simulink model "sim_main_esb_2"  (R2018b)
settings: Solver=VariableStepAuto  StartTime=0.0  StopTime=10  RelTol=1e-3
values from neighbouring files (symbols this model uses):
  A = 0.914    [KALMAN.m]    (also in main_cntl.m = eval(A_eq); main_sys.m = double(A_lin); main_sys_klm.m = double(A_lin); main_tf_0.m = A)
  B = 0.25    [KALMAN.m]    (also in main_cntl.m = eval(B_eq); main_sys.m = double(B_lin); main_sys_klm.m = double(B_lin); main_tf_1.m = eval(B))
  bm = 0.4e-3    (= 0.0004)    [main_cntl.m]    (also in main_sys.m = 0.00047698; main_sys_klm.m = 0.00047698; main_tf_1.m; main_tf_10.m = 0.00047698)
  C = 0.344    [KALMAN.m]    (also in main_sys.m = double( subs( C) ); main_sys_klm.m = double( subs( C) ); main_tf_0.m = [ 0 , 0  , Ks , ds , -Ks , -ds, 0 ]; main_tf_1.m = C_mes)
  D = zeros(7,2)    [main_sys.m]    (also in main_sys_klm.m = zeros(2,2); main_tf_0.m = [ 0 , 0 ]; main_tf_1.m = zeros(1,1); main_tf_10.m = zeros(2,2))
  dg = 0.65    [main_cntl.m]    (also in main_sys.m; main_sys_klm.m; main_tf_1.m; main_tf_10.m)
  dgs = 6    [main_cntl.m]    (also in main_sys.m; main_sys_klm.m; main_tf_1.m; main_tf_10.m)
  J_act = [0.000306 +  0.28200e-04]    [main_cntl.m]    (also in main_sys.m; main_sys_klm.m; main_tf_1.m; main_tf_10.m)
  Js_int = 1.1e-4    (= 0.00011)    [main_cntl.m]    (also in main_sys.m; main_sys_klm.m; main_tf_1.m; main_tf_10.m)
  Kg = 2.7e4    (= 27000)    [main_cntl.m]    (also in main_sys.m; main_sys_klm.m; main_tf_1.m; main_tf_10.m)
  rg = 160    [main_cntl.m]    (also in main_sys.m; main_sys_klm.m; main_tf_1.m; main_tf_10.m)
  Vel_mot_nom = 263    [main_cntl.m]    (also in main_sys.m; main_sys_klm.m; main_tf_1.m; main_tf_10.m)
settings Model: Creator=eshojaei  LastModifiedBy=eshojaei

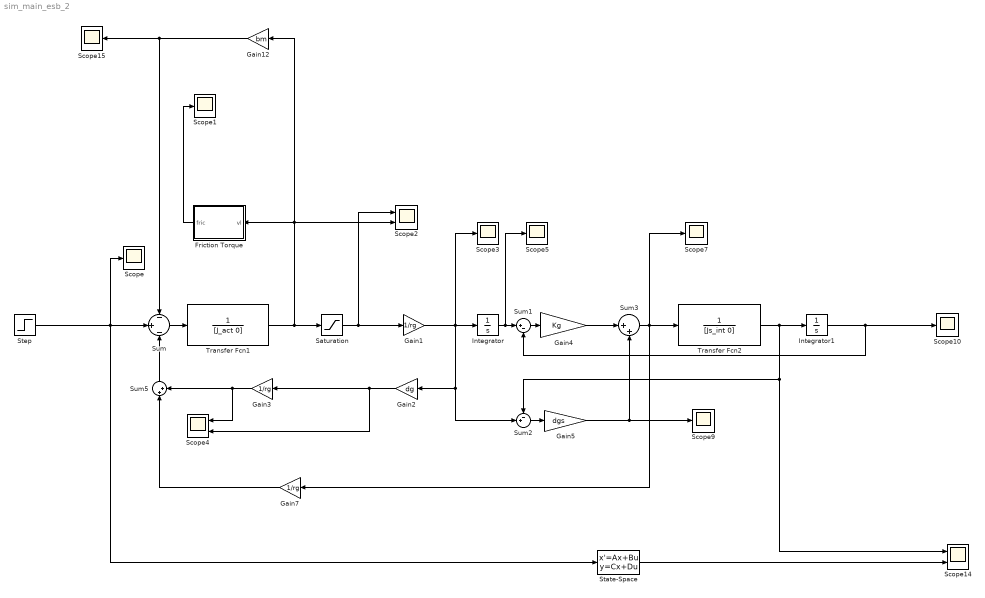
== system sim_main_esb_2 ==
  Friction Torque : MATLAB Function  TreatAsAtomicUnit=on
  Gain1 : Gain  Gain=1/rg
  Gain12 : Gain  Gain=bm
  Gain2 : Gain  Gain=dg
  Gain3 : Gain  Gain=1/rg
  Gain4 : Gain  Gain=Kg
  Gain5 : Gain  Gain=dgs
  Gain7 : Gain  Gain=1/rg
  Integrator : Integrator
  Integrator1 : Integrator
  Saturation : Saturate  UpperLimit=Vel_mot_nom  LowerLimit=-Vel_mot_nom
  Scope{,1,3,5,7,9..10,15} (8 alike) : Scope
  Scope14 : Scope  NumInputPorts=2
  Scope2 : Scope  NumInputPorts=2
  Scope4 : Scope  NumInputPorts=2
  State-Space : StateSpace  A=A  B=B  C=C  D=D  InitialCondition=0
  Step : Step  Time=.1  After=.1  SampleTime=0
  Sum : Sum  Inputs=-|+|-
  Sum1 : Sum  Inputs=|+-
  Sum2 : Sum  Inputs=-+|
  Sum3 : Sum  Inputs=|++
  Sum5 : Sum  Inputs=|++
  Transfer Fcn1 : TransferFcn  Denominator=[J_act 0]
  Transfer Fcn2 : TransferFcn  Denominator=[Js_int 0]
  wires:
  Sum/1 -> Transfer Fcn1/1
  Transfer Fcn1/1 -> Saturation/1, Gain12/1, Friction Torque/1(vl), Scope2/2
  Transfer Fcn2/1 -> Integrator1/1, Scope14/1, Sum2/1
  Gain7/1 -> Sum5/1
  Step/1 -> State-Space/1, Scope/1, Sum/2
  Integrator/1 -> Sum1/1, Scope5/1
  Sum1/1 -> Gain4/1
  Sum5/1 -> Sum/3
  Sum3/1 -> Gain7/1, Transfer Fcn2/1, Scope7/1
  Gain5/1 -> Sum3/2, Scope9/1
  Gain2/1 -> Scope4/2, Gain3/1
  Saturation/1 -> Gain1/1, Scope2/1
  Gain1/1 -> Scope3/1, Integrator/1, Sum2/2, Gain2/1
  Gain3/1 -> Sum5/2, Scope4/1
  Sum2/1 -> Gain5/1
  State-Space/1 -> Scope14/2
  Gain12/1 -> Sum/1, Scope15/1
  Friction Torque/1(fric) -> Scope1/1
  Integrator1/1 -> Sum1/2, Scope10/1
  Gain4/1 -> Sum3/1

== matlab function sim_main_esb_2/Friction Torque ==
  data: vl input; fric output
function fric = fcn(vl)

    
   fric = (5981672325465929*vl)/147573952589676412928 + (7059617857129123*tanh((6072588977179245*vl)/36028797018963968))/144115188075855872 + (2558104915892175*tanh((5176012883402097*vl)/576460752303423488))/72057594037927936;
